simulink model "igbt_design"  (Simulink 9.1)
settings: Solver=VariableStepAuto  StartTime=0.0  StopTime=10.0  RelTol=1e-3
libraries: powerlib x12, simulink x1
settings Model: Creator=Anoop  LastModifiedBy=Anoop
settings DataIOCC: SaveFormat=Dataset
settings OptimizationCC: LifeSpan=auto
settings DebuggingCC: UnderspecifiedInitializationDetection=Simplified  MergeDetectMultiDrivingBlocksExec=error  SFUnexpectedBacktrackingDiag=error  SFNoUnconditionalDefaultTransitionDiag=error  SFExecutionAtInitializationDiag=warning
settings HardwareCC: ProdBitPerPointer=64  ProdBitPerSizeT=64  ProdBitPerPtrDiffT=64  ProdLargestAtomicFloat=Float  ProdIntDivRoundTo=Zero  ProdEndianess=LittleEndian  ProdWordSize=64  ProdHWDeviceType=Intel->x86-64 (Windows64)
settings ModelReferenceCC: PropagateSignalLabelsOutOfModel=on
settings CodeAppCC: StateflowObjectComments=off
settings GRTTargetCC: TargetLangStandard=C99 (ISO)  CombineOutputUpdateFcns=on  GRTInterface=off
settings ConfigComp: CovMetricSettings=dwe  CovHtmlReporting=off  CovSaveCumulativeToWorkspaceVar=off  CovSaveSingleToWorkspaceVar=off  CovExternalEMLEnable=on

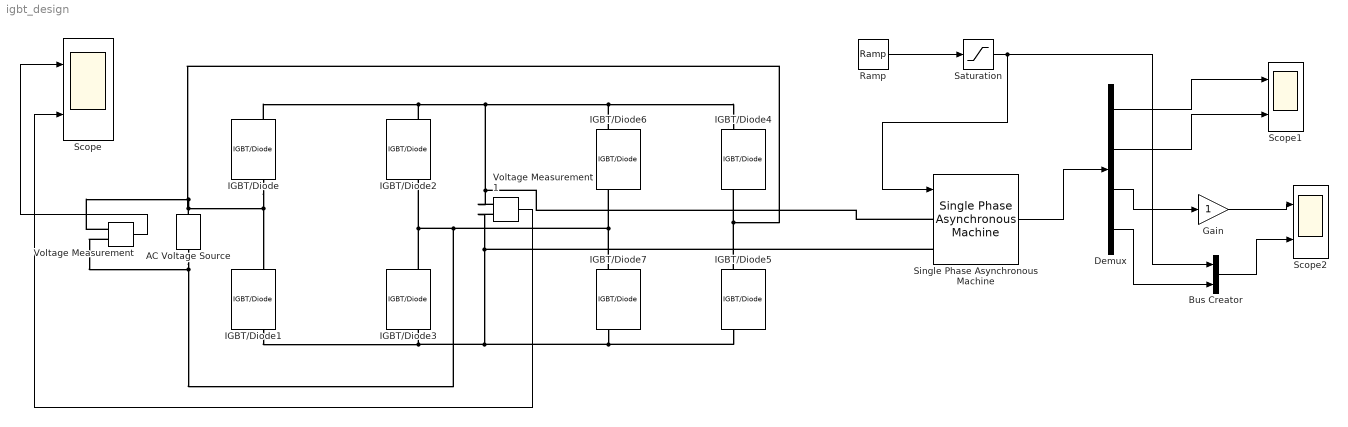
== system igbt_design ==
  AC Voltage Source : powerlib/Electrical Sources/AC Voltage Source  Amplitude=220  Phase=0  Frequency=60  SampleTime=0  Measurements=None  BusType=swing  Pref=10e3  Qref=0  Qmin=-inf  Qmax=+inf
  Bus Creator : BusCreator  Inputs=2
  Demux : Demux
  Gain : Gain
  IGBT/Diode{,1..7} (8 alike) : powerlib/Power Electronics/IGBT//Diode  Ron=1e-3  Rs=1e5  Cs=inf  Measurements=on
  Ramp : simulink/Sources/Ramp  slope=1  start=0  InitialOutput=0
  Saturation : Saturate
  Scope : Scope  NumInputPorts=2
  Scope1 : Scope  NumInputPorts=2
  Scope2 : Scope  NumInputPorts=2
  Single Phase Asynchronous Machine : powerlib/Machines/Single Phase Asynchronous Machine  MechanicalLoad=Torque Tm  UNITS=SI  MachineType=Split Phase  MeasurementBus=off  NominalParameters="[ .25*746  110  60]"  MainWindingStator="[2.02  7.4e-3]"  MainWindingRotor="[4.12  5.6e-3]"  MutualInductance=0.1772  AuxiliaryWinding="[7.14  8.5e-3]"  Mechanical="[0.0146  0  2 1.18]"  CapacitorStart="[2  254.7e-6]"  CapacitorRun="[18  21.1e-6]"  DisconnectionSpeed=75  InitialSpeed=0  DataType=SI  TsPowergui=0  TsBlock=-1
      settings: SourceProductName=Simscape Power Systems  SourceProductBaseCode=PS
  Voltage Measurement : powerlib/Measurements/Voltage Measurement  PhasorSimulation=off  OutputType=Complex  PSBequivalent=0
  Voltage Measurement1 : powerlib/Measurements/Voltage Measurement  PhasorSimulation=off  OutputType=Complex  PSBequivalent=0
  wires:
  Ramp/1 -> Saturation/1
  Voltage Measurement1/1 -> Scope/2
  Voltage Measurement/1 -> Scope/1
  Saturation/1 -> Bus Creator/1, Single Phase Asynchronous Machine/1
  Single Phase Asynchronous Machine/1 -> Demux/1
  Demux/2 -> Scope1/2
  Demux/1 -> Scope1/1
  Demux/4 -> Bus Creator/2
  Demux/3 -> Gain/1
  Gain/1 -> Scope2/1
  Bus Creator/1 -> Scope2/2
  connections:
  IGBT/Diode7/LConn1 -- IGBT/Diode6/RConn1 -- Voltage Measurement/LConn2 -- AC Voltage Source/LConn1 -- IGBT/Diode3/RConn1 -- IGBT/Diode2/LConn1
  IGBT/Diode5/LConn1 -- Voltage Measurement/LConn1 -- AC Voltage Source/RConn1 -- IGBT/Diode1/RConn1 -- IGBT/Diode/LConn1 -- IGBT/Diode4/RConn1
  IGBT/Diode1/LConn1 -- IGBT/Diode7/RConn1 -- IGBT/Diode5/RConn1 -- Voltage Measurement1/LConn2 -- Single Phase Asynchronous Machine/LConn2 -- IGBT/Diode3/LConn1
  IGBT/Diode6/LConn1 -- Single Phase Asynchronous Machine/LConn1 -- Voltage Measurement1/LConn1 -- IGBT/Diode2/RConn1 -- IGBT/Diode/RConn1 -- IGBT/Diode4/LConn1
